simulink model "mdl_VD_FirstOrderEngineModel_R2024a_SLX"  (R2024a)
settings: Solver=ode4  StartTime=startTime  StopTime=endTime  FixedStep=deltaT  MaxStep=deltaT  RelTol=1e-3  EnableMultiTasking=on
values from neighbouring files (symbols this model uses):
  initialStates = 0    [script_test_fcn_VD_FirstOrderEngineModelSimulink.m]
undefined symbols (not defined in the file or in its folder): parameters
settings Model: Creator=snb10  LastModifiedBy=snb10
settings SolverCC: AlgebraicLoopSolver=TrustRegion
settings DataIOCC: LimitDataPoints=on  SaveFormat=Array  SignalLoggingSaveFormat=ModelDataLogs  SaveOutput=off  SignalLogging=off  DSMLogging=off  SaveTime=off  SignalLoggingName=sigsOut
settings OptimizationCC: InitFltsAndDblsToZero=on  LifeSpan=inf
settings DebuggingCC: SaveWithParameterizedLinksMsg=none  UnderspecifiedInitializationDetection=Classic  MergeDetectMultiDrivingBlocksExec=none  SignalResolutionControl=TryResolveAllWithWarning  MultiTaskDSMMsg=warning  MultiTaskCondExecSysMsg=none  FcnCallInpInsideContextMsg=warning  UnconnectedInputMsg=warning  UnconnectedOutputMsg=warning  UnconnectedLineMsg=warning  StateNameClashWarn=warning  SFUnexpectedBacktrackingDiag=warning  SFNoUnconditionalDefaultTransitionDiag=warning  SFExecutionAtInitializationDiag=none  ArithmeticOperatorsInVariantConditions=warning
settings HardwareCC: ProdBitPerPointer=32  ProdBitPerSizeT=32  ProdBitPerPtrDiffT=32  ProdLargestAtomicFloat=None  ProdIntDivRoundTo=Undefined  ProdEndianess=Unspecified  ProdWordSize=32  ProdHWDeviceType=32-bit Generic  TargetUnknown=on
settings ModelReferenceCC: EnableRefExpFcnMdlSchedulingChecks=on  PropagateSignalLabelsOutOfModel=off
settings SFSimCC: SimUseLocalCustomCode=off  CustomCodeUndefinedFunction=UseInterfaceOnly
settings RTWCC: RTWUseLocalCustomCode=off  GPUComputeCapability=3.5  DLArmComputeVersion=19.05
settings CodeAppCC: StateflowObjectComments=on
settings GRTTargetCC: TargetFcnLib=ansi_tfl_tmw.mat  TargetLangStandard=C89/C90 (ANSI)  CombineOutputUpdateFcns=off  GRTInterface=on
settings ConfigComp: CovMetricSettings=dw  CovSaveCumulativeToWorkspaceVar=on  CovSaveSingleToWorkspaceVar=on  CovExternalEMLEnable=off  CovBoundaryAbsTol=1.0e-5

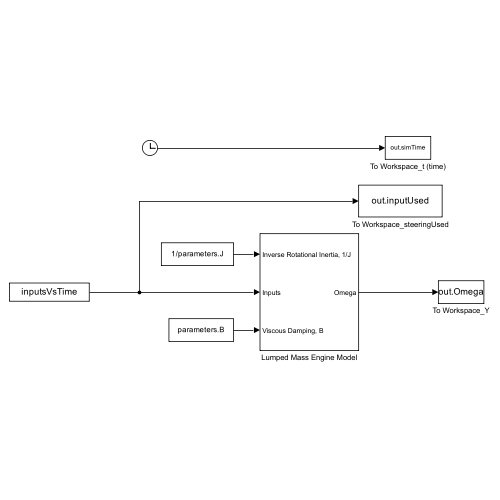
[thumbnail: Simulink's stored preview of the top-level diagram]
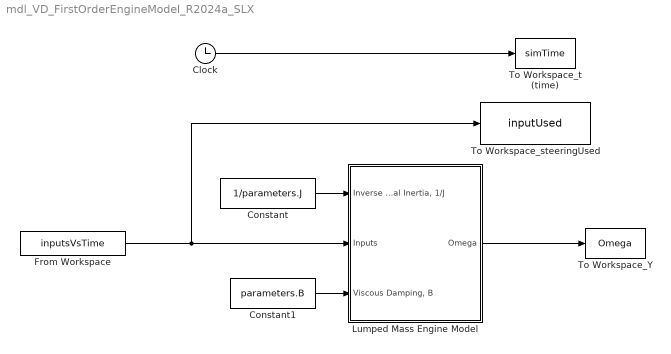
== system mdl_VD_FirstOrderEngineModel_R2024a_SLX ==
  Clock : Clock
  Constant : Constant  Value=1/parameters.J  SampleTime=.01
  Constant1 : Constant  Value=parameters.B  SampleTime=.01
  From Workspace : FromWorkspace  VariableName=inputsVsTime  OutDataTypeStr=double  SampleTime=.01  OutputAfterFinalValue=Holding final value
  Lumped Mass Engine Model : Subsystem
  To Workspace_Y : ToWorkspace  VariableName=Omega  SampleTime=.01
  To Workspace_steeringUsed : ToWorkspace  VariableName=inputUsed  SampleTime=.01
  To Workspace_t (time) : ToWorkspace  VariableName=simTime  SampleTime=.01
  wires:
  Clock/1 -> To Workspace_t (time)/1
  Lumped Mass Engine Model/1(Omega) -> To Workspace_Y/1
  From Workspace/1 -> Lumped Mass Engine Model/2(Inputs), To Workspace_steeringUsed/1
  Constant/1 -> Lumped Mass Engine Model/1("Inverse Rotational Inertia, 1/J")
  Constant1/1 -> Lumped Mass Engine Model/3("Viscous Damping, B")

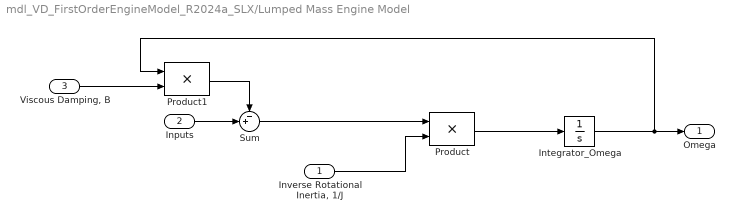
== system mdl_VD_FirstOrderEngineModel_R2024a_SLX/Lumped Mass Engine Model ==
  "Inverse Rotational Inertia, 1/J" : Inport
  Inputs : Inport  Port=2
  "Viscous Damping, B" : Inport  Port=3
  Integrator_Omega : Integrator  InitialCondition=initialStates(1)
  Product : Product  SaturateOnIntegerOverflow=on  OutDataTypeStr=Inherit: Same as first input
  Product1 : Product  SaturateOnIntegerOverflow=on  OutDataTypeStr=Inherit: Same as first input
  Sum : Sum  Inputs=-+|
  Omega : Outport
  wires:
  Integrator_Omega/1 -> Product1/1, Omega/1
  Product/1 -> Integrator_Omega/1
  "Inverse Rotational Inertia, 1/J"/1 -> Product/2
  "Viscous Damping, B"/1 -> Product1/2
  Product1/1 -> Sum/1
  Inputs/1 -> Sum/2
  Sum/1 -> Product/1
